simulink model "W05_P1"  (R2024b)
settings: Solver=ode4  StartTime=0  StopTime=T_final  FixedStep=h  RelTol=1e-3
values from neighbouring files (symbols this model uses):
  x0 = zeros(12,1);  x0(8) = V.y0    [W05_check.m]
undefined symbols (not defined in the file or in its folder): beta_c, k_neg, k_pos, Kd, Kp, mp, n_max, n_min, rp, V_c, X_ff, y_pont
settings Model: Creator=admin  LastModifiedBy=admin
settings DataIOCC: ReturnWorkspaceOutputs=off

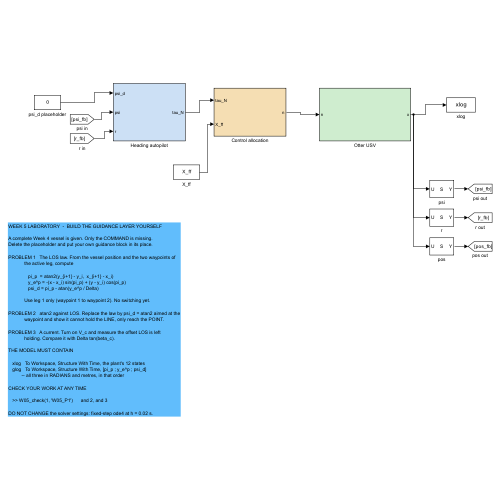
[thumbnail: Simulink's stored preview of the top-level diagram]
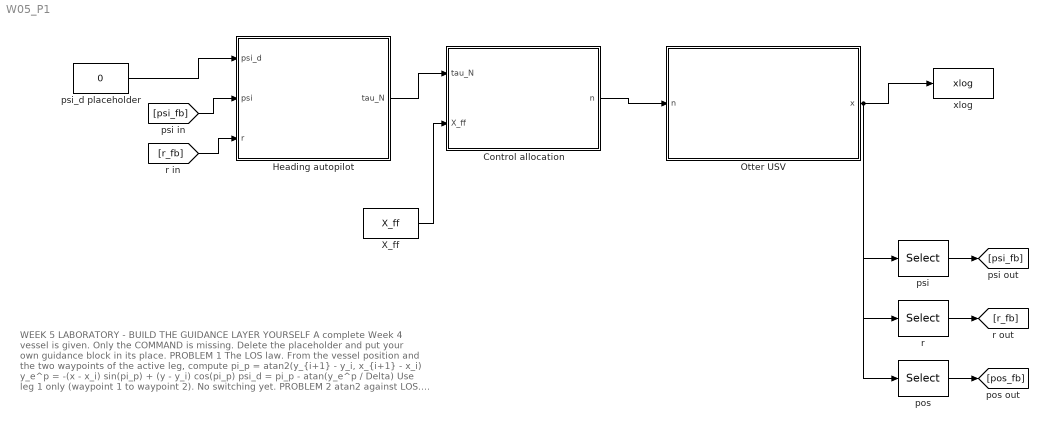
== system W05_P1 ==
  note: WEEK 5 LABORATORY  -  BUILD THE GUIDANCE LAYER YOURSELF
      |
      | A complete Week 4 vessel is given. Only the COMMAND is missing.
      | Delete the placeholder and put your own guidance block in its place.
      |
      | PROBLEM 1   The LOS law. From the vessel position and the two waypoints of
      |             the active leg, compute
      |
      |                pi_p  = atan2(y_{i+1} - y_i,  x_{i+1} - x_i)
      |                y_e^p = -(x - x_i) sin(pi_p) + (y - y_i) cos(pi_p)
      |                psi_d = pi_p - atan(y_e^p / Delta)
      |
      |             Use leg 1 only (waypoint 1 to waypoint 2). No switching yet.
      |
      | PROBLEM 2   atan2 against LOS. Replace the law by psi_d = atan2 aimed at the
      |             waypoint and show it cannot hold the LINE, only reach the POINT.
      |
      | PROBLEM 3   A current. Turn on V_c and measure the offset LOS is left
      |             holding. Compare it with Delta tan(beta_c).
      |
      | THE MODEL MUST CONTAIN
      |
      |    xlog   To Workspace, Structure With Time, the plant's 12 states
      |    glog   To Workspace, Structure With Time, [pi_p ; y_e^p ; psi_d]
      |           -- all three in RADIANS and metres, in that order
      |
      | CHECK YOUR WORK AT ANY TIME
      |
      |    >> W05_check(1, 'W05_P1')      and 2, and 3
      |
      | DO NOT CHANGE the solver settings: fixed-step ode4 at h = 0.02 s.
  Control allocation : Subsystem
  Heading autopilot : Subsystem
  Otter USV : Subsystem
  X_ff : Constant  Value=X_ff
  pos : Selector  InputPortWidth=12  IndexOptions=Index vector (dialog)  Indices=[7 8]  OutputSizes=1
  psi : Selector  InputPortWidth=12  IndexOptions=Index vector (dialog)  Indices=12  OutputSizes=1
  psi_d placeholder : Constant  Value=0
  r : Selector  InputPortWidth=12  IndexOptions=Index vector (dialog)  Indices=6  OutputSizes=1
  xlog : ToWorkspace  VariableName=xlog  SaveFormat=Structure With Time  SampleTime=-1
  wires:
  Heading autopilot/1(tau_N) -> Control allocation/1(tau_N)
  X_ff/1 -> Control allocation/2(X_ff)
  Control allocation/1(n) -> Otter USV/1(n)
  Otter USV/1(x) -> xlog/1, psi/1, r/1, pos/1
  psi/1 -> [psi_fb]
  r/1 -> [r_fb]
  [psi_fb] -> Heading autopilot/2(psi)
  [r_fb] -> Heading autopilot/3(r)
  pos/1 -> [pos_fb]
  psi_d placeholder/1 -> Heading autopilot/1(psi_d)

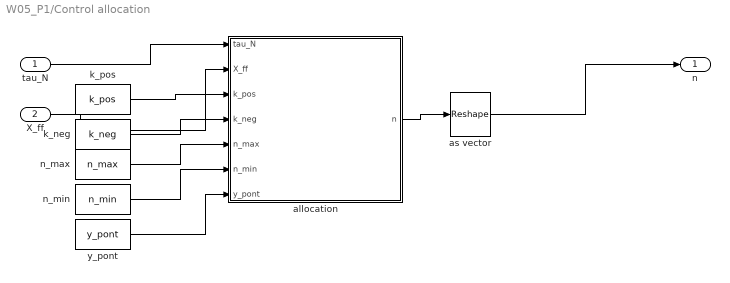
== system W05_P1/Control allocation ==
  tau_N : Inport
  X_ff : Inport  Port=2
  allocation : MATLAB Function  TreatAsAtomicUnit=on
  as vector : Reshape
  k_neg : Constant  Value=k_neg
  k_pos : Constant  Value=k_pos
  n_max : Constant  Value=n_max
  n_min : Constant  Value=n_min
  y_pont : Constant  Value=y_pont
  n : Outport
  wires:
  k_pos/1 -> allocation/3(k_pos)
  k_neg/1 -> allocation/4(k_neg)
  n_max/1 -> allocation/5(n_max)
  n_min/1 -> allocation/6(n_min)
  y_pont/1 -> allocation/7(y_pont)
  tau_N/1 -> allocation/1(tau_N)
  X_ff/1 -> allocation/2(X_ff)
  allocation/1(n) -> as vector/1
  as vector/1 -> n/1

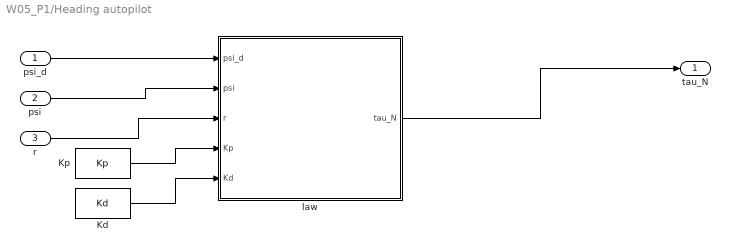
== system W05_P1/Heading autopilot ==
  psi_d : Inport
  psi : Inport  Port=2
  r : Inport  Port=3
  Kd : Constant  Value=Kd
  Kp : Constant  Value=Kp
  law : MATLAB Function  TreatAsAtomicUnit=on
  tau_N : Outport
  wires:
  Kp/1 -> law/4(Kp)
  Kd/1 -> law/5(Kd)
  psi_d/1 -> law/1(psi_d)
  psi/1 -> law/2(psi)
  r/1 -> law/3(r)
  law/1(tau_N) -> tau_N/1

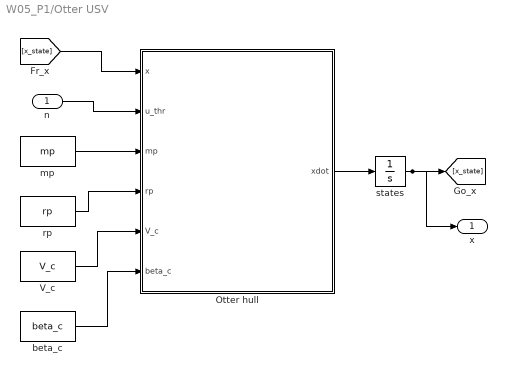
== system W05_P1/Otter USV ==
  n : Inport
  Otter hull : MATLAB Function  TreatAsAtomicUnit=on
  V_c : Constant  Value=V_c
  beta_c : Constant  Value=beta_c
  mp : Constant  Value=mp
  rp : Constant  Value=rp
  states : Integrator  InitialCondition=x0
  x : Outport
  wires:
  states/1 -> x/1, [x_state]
  Otter hull/1(xdot) -> states/1
  [x_state] -> Otter hull/1(x)
  beta_c/1 -> Otter hull/6(beta_c)
  n/1 -> Otter hull/2(u_thr)
  mp/1 -> Otter hull/3(mp)
  rp/1 -> Otter hull/4(rp)
  V_c/1 -> Otter hull/5(V_c)

== matlab function W05_P1/Control allocation/allocation ==
  data: tau_N input; n output double size=[2 1]; X_ff input; k_pos input; k_neg input; n_max input; n_min input; y_pont input
function n = allocation(tau_N, X_ff, k_pos, k_neg, n_max, n_min, y_pont)
%#codegen
% Demanded surge force and yaw moment to two shaft speeds. Appendix A1.
T = [X_ff/2 + tau_N/(2*y_pont);
     X_ff/2 - tau_N/(2*y_pont)];
n = zeros(2,1);
for i = 1:2
    if T(i) >= 0
        ni =  sqrt( T(i) / k_pos);
    else
        ni = -sqrt(-T(i) / k_neg);
    end
    n(i) = min(max(ni, n_min), n_max);
end
end

== matlab function W05_P1/Heading autopilot/law ==
  data: psi_d input; tau_N output double size=[1 1]; psi input; r input; Kp input; Kd input
function tau_N = law(psi_d, psi, r, Kp, Kd)
%#codegen
%LAW  Week 4's heading autopilot, unchanged.
%
%  tau_N = Kp ssa(psi_d - psi) - Kd r
%
%  The wrap is not optional here: guidance produces commands anywhere in
%  (-pi, pi], so the +-180 deg seam is crossed on almost every mission.
e = mod(psi_d - psi + pi, 2*pi) - pi;
tau_N = Kp*e - Kd*r;

== matlab function W05_P1/Otter USV/Otter hull ==
  data: x input; xdot output double size=[12 1]; u_thr input; mp input; rp input; V_c input; beta_c input
function xdot = otter_hull(x, u_thr, mp, rp, V_c, beta_c)
% Fossen's otter.m, called unchanged from Tools/MSS/VESSELS.
%
%   x       12 states, fed back from the integrator
%   u_thr   propeller shaft speeds [rad/s]
%
% otter.m is not written for code generation, so the call is extrinsic and
% xdot has to be pre-sized for Simulink to know the output width.
coder.extrinsic('otter');

xdot = zeros(12,1);
xdot = otter(x, u_thr, mp, rp, V_c, beta_c);
end
